simulink model "matlab2014a_foc_test_0423"  (R2014a)
settings: Solver=ode45  StartTime=0.0  StopTime=5  RelTol=1e-3
settings Model: Creator=ruanpei  LastModifiedBy=ruanpei

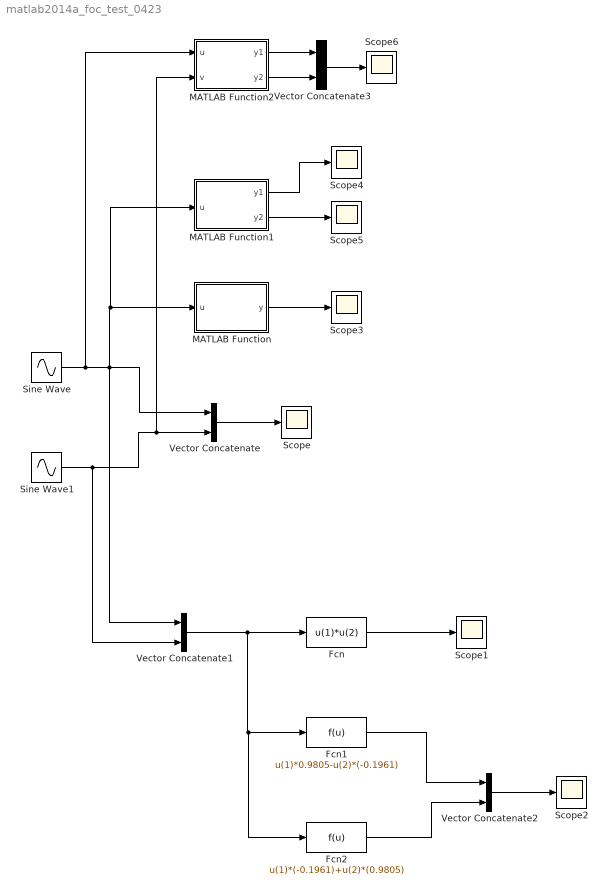
== system matlab2014a_foc_test_0423 ==
  Fcn : Fcn  Expr=u(1)*u(2)
  Fcn1 : Fcn  Expr=u(1)*0.9805-u(2)*(-0.1961)
  Fcn2 : Fcn  Expr=u(1)*(-0.1961)+u(2)*(0.9805)
  MATLAB Function : MATLAB Function  TreatAsAtomicUnit=on
  MATLAB Function1 : MATLAB Function  TreatAsAtomicUnit=on
  MATLAB Function2 : MATLAB Function  TreatAsAtomicUnit=on
  Scope{,1..6} (7 alike) : Scope
      Scope2 settings: SaveName=ScopeData2
      Scope3 settings: SaveName=ScopeData3
      Scope4 settings: SaveName=ScopeData4
      Scope5 settings: SaveName=ScopeData5
      Scope6 settings: SaveName=ScopeData6
  Sine Wave : Sin  Frequency=50  SampleTime=50e-6
  Sine Wave1 : Sin  Frequency=50  Phase=0.5*pi  SampleTime=50e-6
  Vector Concatenate{,1..3} (4 alike) : Concatenate
  wires:
  Sine Wave/1 -> MATLAB Function2/1(u), MATLAB Function1/1(u), MATLAB Function/1(u), Vector Concatenate1/1, Vector Concatenate/1
  Vector Concatenate/1 -> Scope/1
  Vector Concatenate1/1 -> Fcn2/1, Fcn1/1, Fcn/1
  Sine Wave1/1 -> Vector Concatenate1/2, MATLAB Function2/2(v), Vector Concatenate/2
  Fcn/1 -> Scope1/1
  Fcn1/1 -> Vector Concatenate2/1
  Vector Concatenate2/1 -> Scope2/1
  Fcn2/1 -> Vector Concatenate2/2
  MATLAB Function/1(y) -> Scope3/1
  MATLAB Function1/1(y1) -> Scope4/1
  MATLAB Function1/2(y2) -> Scope5/1
  MATLAB Function2/1(y1) -> Vector Concatenate3/1
  MATLAB Function2/2(y2) -> Vector Concatenate3/2
  Vector Concatenate3/1 -> Scope6/1

== matlab function matlab2014a_foc_test_0423/MATLAB Function1 ==
  data: u input; y1 output; y2 output
function [y1,y2] = fcn(u)
%#codegen

y1 = sin(u);
y2 = cos(u)*sin(u);

== matlab function matlab2014a_foc_test_0423/MATLAB Function ==
  data: u input; y output
function y = fcn(u)
%#codegen

y = sin(u);

== matlab function matlab2014a_foc_test_0423/MATLAB Function2 ==
  data: u input; y1 output; y2 output; v input
function [y1,y2] = fcn(u,v)
%#codegen

y1 = sin(u);
y2 = cos(u)*sin(v);
